simulink model "MagLev_1DOF_Slice_with_noise"  (R2020b)
settings: Solver=ode45  StartTime=0.0  StopTime=15  FixedStep=1e-5  RelTol=1e-3
values from neighbouring files (symbols this model uses):
  c = 0.005    [setup.m]
  caseNumber = 2    [setup.m]
  chi_0 = 0    [setup.m]
  dY_0 = 0.5    [setup.m]
  epsilon = 1e-3    (= 0.001)    [setup.m]
  eth10 = 0.0001    [setup.m]
  g = 9.81    [setup.m]
  gamma_ALCOS = 1000    [setup.m]
  gamma_s = 10    [setup.m]
  gamma_SLICE = 100    [setup.m]
  gamma_y = 10    [setup.m]
  k = 1    [setup.m]
  k0 = kk^3    (= 1000)    [setup.m]
  k1 = 3*kk^2    (= 300)    [setup.m]
  k2 = 3*kk    (= 30)    [setup.m]
  lambda_0 = -0.02    [setup.m]
  m = 0.0844    [setup.m]
  mu = 10    [setup.m]
  nu = 1    [setup.m]
  Omega = [ ... (first row only)    [setup.m]
  R = 2.52    [setup.m]
  s = [1; 2; 10; 20; 5; 7]    [setup.m]
  tt1 = 1    [setup.m]
  tt2 = 3    [setup.m]
  tt3 = 5    [setup.m]
  tt4 = 7    [setup.m]
  Y_0 = -1    [setup.m]
(part 1 of 2)
settings Model: Creator=Alexey  LastModifiedBy=Sviat
settings DataIOCC: ReturnWorkspaceOutputs=off
settings DebuggingCC: ArithmeticOperatorsInVariantConditions=warning
settings SFSimCC: SimUseLocalCustomCode=off  CustomCodeUndefinedFunction=UseInterfaceOnly
settings RTWCC: RTWUseLocalCustomCode=off
settings CodeAppCC: StateflowObjectComments=on

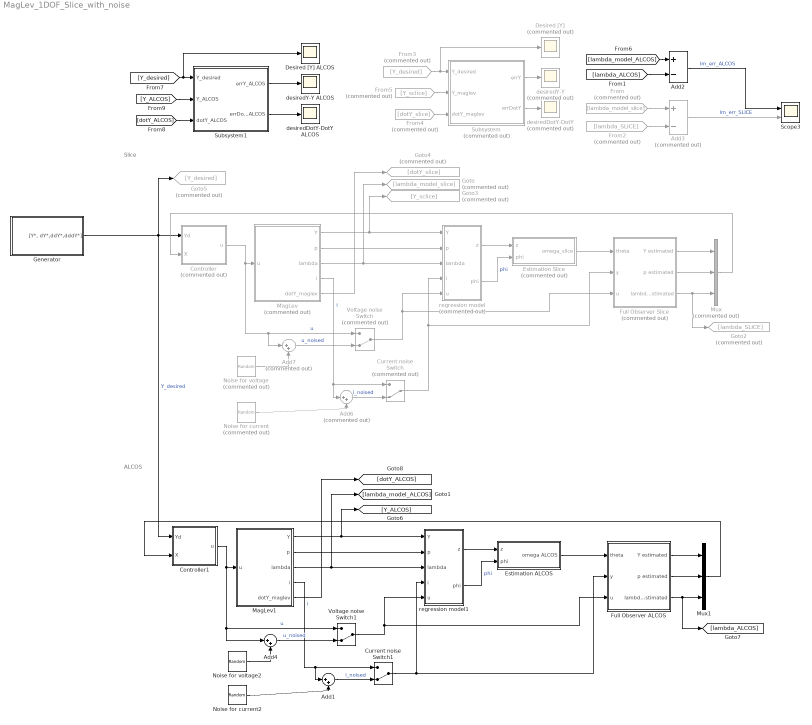
== system MagLev_1DOF_Slice_with_noise ==
  note: Slice
  note: ALCOS
  Add1 : Sum  Inputs=|++
  Add2 : Sum  Inputs=+-
  Add3 : Sum  Commented=on  Inputs=+-
  Add4 : Sum  Inputs=|++
  Add6 : Sum  Commented=on  Inputs=|++
  Add7 : Sum  Commented=on  Inputs=|++
  Controller : MATLAB Function  Commented=on  TreatAsAtomicUnit=on
  Controller1 : MATLAB Function  TreatAsAtomicUnit=on
  Current noise Switch : ManualSwitch  Commented=on  CurrentSetting=0
  Current noise Switch1 : ManualSwitch  CurrentSetting=0
  Desired [Y] : Scope  Commented=on
  Desired [Y] ALCOS : Scope
  Estimation ALCOS : Subsystem
  Estimation Slice : Subsystem  Commented=on
  From : From  Commented=on  GotoTag=lambda_model_slice
  From2 : From  Commented=on  GotoTag=lambda_SLICE
  From3 : From  Commented=on  GotoTag=Y_desired
  From4 : From  Commented=on  GotoTag=dotY_slice
  From5 : From  Commented=on  GotoTag=Y_sclice
  Full Observer ALCOS : Subsystem
  Full Observer Slice : Subsystem  Commented=on
  Generator : Subsystem
  Goto : Goto  Commented=on  GotoTag=lambda_model_slice
  Goto2 : Goto  Commented=on  GotoTag=lambda_SLICE
  Goto3 : Goto  Commented=on  GotoTag=Y_sclice
  Goto4 : Goto  Commented=on  GotoTag=dotY_slice
  Goto5 : Goto  Commented=on  GotoTag=Y_desired
  MagLev : Subsystem  Commented=on
  MagLev1 : Subsystem
  Mux : Mux  Commented=on  Inputs=3
  Mux1 : Mux  Inputs=3
  Noise for current : UniformRandomNumber  Commented=on  Minimum=-0.01  Maximum=0.01  SampleTime=0.0001
  Noise for current2 : UniformRandomNumber  Minimum=-0.01  Maximum=0.01  SampleTime=0.0001
  Noise for voltage : UniformRandomNumber  Commented=on  Minimum=-0.1  Maximum=0.1  SampleTime=0.0001
  Noise for voltage2 : UniformRandomNumber  Minimum=-0.1  Maximum=0.1  SampleTime=0.0001
  Scope3 : Scope  NumInputPorts=2
  Subsystem : Subsystem  Commented=on
  Subsystem1 : Subsystem
  Voltage noise Switch : ManualSwitch  Commented=on  CurrentSetting=0
  Voltage noise Switch1 : ManualSwitch  CurrentSetting=0
  desiredDotY-DotY : Scope  Commented=on
  desiredDotY-DotY ALCOS : Scope
  desiredY-Y : Scope  Commented=on
  desiredY-Y ALCOS : Scope
  regression model : Subsystem  Commented=on
  regression model1 : Subsystem
  wires:
  Controller/1(u) -> MagLev/1(u), Add7/1, Voltage noise Switch/1  "u"
  regression model/2(phi) -> Estimation Slice/2(phi)  "phi"
  regression model/1(z) -> Estimation Slice/1(z)
  MagLev/4(i) -> Add6/1, Current noise Switch/1  "i"
  Estimation Slice/1(omega_slice) -> Full Observer Slice/1(theta)
  From/1 -> Add3/1
  [lambda_ALCOS] -> Add2/2
  From2/1 -> Add3/2
  Add3/1 -> Scope3/2  "lm_err_SLICE"
  Current noise Switch/1 -> Full Observer Slice/2(y), regression model/4(i)
  Noise for voltage/1 -> Add7/2
  Noise for current/1 -> Add6/2
  Add6/1 -> Current noise Switch/2  "i_noised"
  Add7/1 -> Voltage noise Switch/2  "u_noised"
  Voltage noise Switch/1 -> Full Observer Slice/3(u), regression model/5(u)
  Subsystem/1(errY) -> desiredY-Y/1
  Subsystem/2(errDotY) -> desiredDotY-DotY/1
  From3/1 -> Desired [Y]/1, Subsystem/1(Y_desired)
  MagLev/1(Y) -> Goto3/1, regression model/1(Y)
  MagLev/2(p) -> regression model/2(p)
  MagLev/3(lambda) -> regression model/3(lambda), Goto/1
  MagLev/5(dotY_maglev) -> Goto4/1
  MagLev1/2(p) -> regression model1/2(p)
  MagLev1/1(Y) -> [Y_ALCOS], regression model1/1(Y)
  Voltage noise Switch1/1 -> Full Observer ALCOS/3(u), regression model1/5(u)
  Add1/1 -> Current noise Switch1/2  "i_noised"
  Noise for voltage2/1 -> Add4/2
  Controller1/1(u) -> MagLev1/1(u), Voltage noise Switch1/1, Add4/1  "u"
  Generator/1("[Y*, dY*,ddY*,dddY*]") -> Goto5/1, Controller/1(Yd), Controller1/1(Yd)  "Y_desired"
  MagLev1/4(i) -> Add1/1, Current noise Switch1/1  "i"
  Current noise Switch1/1 -> Full Observer ALCOS/2(y), regression model1/4(i)
  regression model1/2(phi) -> Estimation ALCOS/2(phi)  "phi"
  regression model1/1(z) -> Estimation ALCOS/1(z)
  Estimation ALCOS/1(omega ALCOS) -> Full Observer ALCOS/1(theta)
  Add4/1 -> Voltage noise Switch1/2  "u_noised"
  MagLev1/3(lambda) -> [lambda_model_ALCOS], regression model1/3(lambda)
  Full Observer Slice/1(Y estimated) -> Mux/1
  Full Observer Slice/2(p estimated) -> Mux/2
  Full Observer Slice/3(lambda estimated) -> Goto2/1, Mux/3
  Full Observer ALCOS/1(Y estimated) -> Mux1/1
  Full Observer ALCOS/2(p estimated) -> Mux1/2
  From5/1 -> Subsystem/2(Y_maglev)
  From4/1 -> Subsystem/3(dotY_maglev)
  Add2/1 -> Scope3/1  "lm_err_ALCOS"
  Noise for current2/1 -> Add1/2
  Mux/1 -> Controller/2(X)
  Full Observer ALCOS/3(lambda estimated) -> [lambda_ALCOS], Mux1/3
  Mux1/1 -> Controller1/2(X)
  [lambda_model_ALCOS] -> Add2/1
  MagLev1/5(dotY_maglev) -> [dotY_ALCOS]
  [dotY_ALCOS] -> Subsystem1/3(dotY_ALCOS)
  [Y_ALCOS] -> Subsystem1/2(Y_ALCOS)
  [Y_desired] -> Desired [Y] ALCOS/1, Subsystem1/1(Y_desired)
  Subsystem1/2(errDotY_ALCOS) -> desiredDotY-DotY ALCOS/1
  Subsystem1/1(errY_ALCOS) -> desiredY-Y ALCOS/1

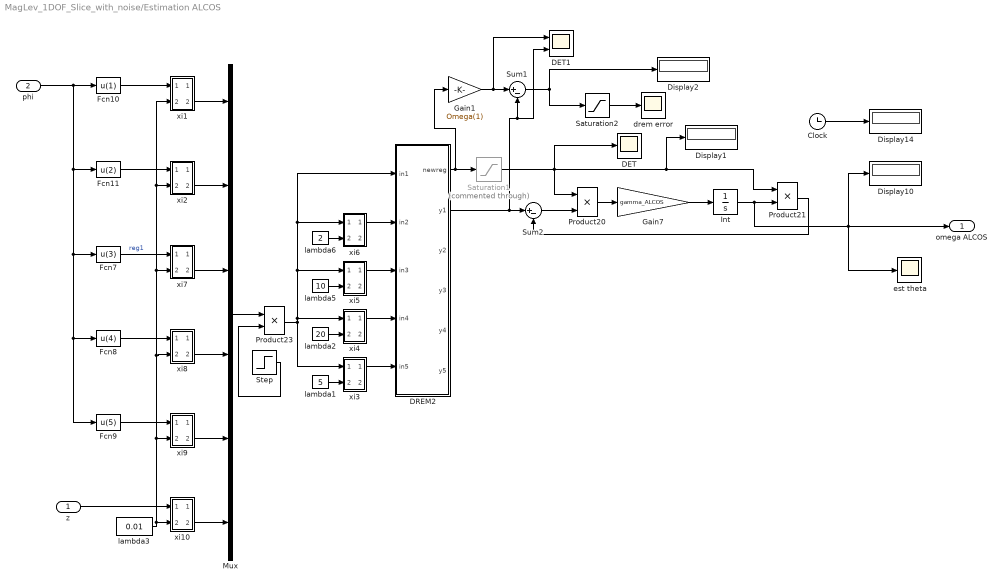
== system MagLev_1DOF_Slice_with_noise/Estimation ALCOS ==
  z : Inport
  phi : Inport  Port=2
  Clock : Clock
  DET : Scope
  DET1 : Scope  NumInputPorts=2
  DREM2 : MATLAB Function  TreatAsAtomicUnit=on
  Display{1..2,10,14} (4 alike) : Display
  Fcn10 : Fcn  Expr=u(1)
  Fcn11 : Fcn  Expr=u(2)
  Fcn7 : Fcn  Expr=u(3)
  Fcn8 : Fcn  Expr=u(4)
  Fcn9 : Fcn  Expr=u(5)
  Gain1 : Gain  Gain=Omega(1)
  Gain7 : Gain  Gain=gamma_ALCOS
  Int : Integrator  InitialCondition=eth10
  Mux : Mux  Inputs=6
  Product20 : Product  RndMeth=Zero
  Product21 : Product  RndMeth=Zero
  Product23 : Product  RndMeth=Zero
  Saturation1 : Saturate  Commented=through  UpperLimit=1000  LowerLimit=-1000
  Saturation2 : Saturate  UpperLimit=1000  LowerLimit=-1000
  Step : Step  Time=0  After=100  SampleTime=0
  Sum1 : Sum  Inputs=|+-
  Sum2 : Sum  Inputs=|+-
  drem error : Scope
  est theta : Scope
  lambda1 : Constant  Value=5
  lambda2 : Constant  Value=20
  lambda3 : Constant  Value=0.01
  lambda5 : Constant  Value=10
  lambda6 : Constant  Value=2
  xi1 : Subsystem
  xi10 : Subsystem
  xi2 : Subsystem
  xi3 : Subsystem
  xi4 : Subsystem
  xi5 : Subsystem
  xi6 : Subsystem
  xi7 : Subsystem
  xi8 : Subsystem
  xi9 : Subsystem
  omega ALCOS : Outport  VectorParamsAs1DForOutWhenUnconnected=off
  wires:
  Mux/1 -> Product23/1
  Product20/1 -> Gain7/1
  Gain7/1 -> Int/1
  Int/1 -> omega ALCOS/1, est theta/1, Display10/1, Product21/2
  Product21/1 -> Sum2/2
  Sum2/1 -> Product20/2
  DREM2/2(y1) -> Sum2/1, DET1/2, Sum1/2
  Clock/1 -> Display14/1
  DREM2/1(newreg) -> Saturation1/1, Gain1/1
  Product23/1 -> DREM2/1(in1), xi6/1(Input), xi5/1(Input), xi4/1(Input), xi3/1(Input)
  lambda1/1 -> xi3/2(lambda)
  xi3/1(Output) -> DREM2/5(in5)
  lambda2/1 -> xi4/2(lambda)
  lambda5/1 -> xi5/2(lambda)
  lambda6/1 -> xi6/2(lambda)
  xi6/1(Output) -> DREM2/2(in2)
  xi5/1(Output) -> DREM2/3(in3)
  xi4/1(Output) -> DREM2/4(in4)
  Fcn9/1 -> xi9/1(Input)
  Fcn8/1 -> xi8/1(Input)
  Fcn7/1 -> xi7/1(Input)  "reg1"
  Fcn11/1 -> xi2/1(Input)
  Fcn10/1 -> xi1/1(Input)
  xi1/2(Output1) -> Mux/1
  xi2/2(Output1) -> Mux/2
  xi7/2(Output1) -> Mux/3
  xi8/2(Output1) -> Mux/4
  xi9/2(Output1) -> Mux/5
  xi10/2(Output1) -> Mux/6
  lambda3/1 -> xi8/2(lambda), xi7/2(lambda), xi1/2(lambda), xi2/2(lambda), xi9/2(lambda), xi10/2(lambda)
  Step/1 -> Product23/2
  Saturation1/1 -> DET/1, Product20/1, Display1/1, Product21/1
  z/1 -> xi10/1(Input)
  phi/1 -> Fcn9/1, Fcn8/1, Fcn7/1, Fcn11/1, Fcn10/1
  Gain1/1 -> DET1/1, Sum1/1
  Sum1/1 -> Display2/1, Saturation2/1
  Saturation2/1 -> drem error/1

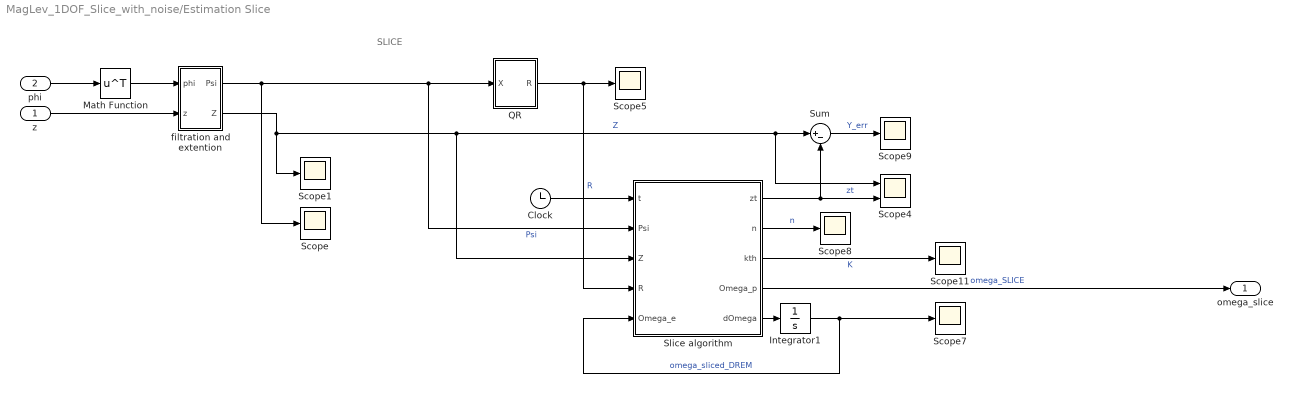
== system MagLev_1DOF_Slice_with_noise/Estimation Slice ==
  note: SLICE
  z : Inport
  phi : Inport  Port=2
  Clock : Clock
  Integrator1 : Integrator  InitialCondition=eth10
  Math Function : Math  Operator=transpose  SignedPower=on  SaturateOnIntegerOverflow=on
  QR : MATLAB Function  TreatAsAtomicUnit=on
  Scope{,1,5,7..9,11} (7 alike) : Scope
  Scope4 : Scope  NumInputPorts=2
  Slice algorithm : MATLAB Function  TreatAsAtomicUnit=on
  Sum : Sum  Inputs=|+-
  filtration and extention : Subsystem
  omega_slice : Outport  VectorParamsAs1DForOutWhenUnconnected=off
  wires:
  z/1 -> filtration and extention/2(z)
  phi/1 -> Math Function/1
  filtration and extention/1(Psi) -> Slice algorithm/2(Psi), QR/1(X), Scope/1  "Psi"
  filtration and extention/2(Z) -> Sum/1, Scope4/1, Slice algorithm/3(Z), Scope1/1  "Z"
  Math Function/1 -> filtration and extention/1(phi)
  Slice algorithm/5(dOmega) -> Integrator1/1
  QR/1(R) -> Scope5/1, Slice algorithm/4(R)  "R"
  Integrator1/1 -> Scope7/1, Slice algorithm/5(Omega_e)  "omega_sliced_DREM"
  Slice algorithm/4(Omega_p) -> omega_slice/1  "omega_SLICE"
  Slice algorithm/1(zt) -> Scope4/2, Sum/2  "zt"
  Slice algorithm/2(n) -> Scope8/1  "n"
  Sum/1 -> Scope9/1  "Y_err"
  Slice algorithm/3(kth) -> Scope11/1  "K"
  Clock/1 -> Slice algorithm/1(t)

== system MagLev_1DOF_Slice_with_noise/Full Observer ALCOS ==
  theta : Inport
  y : Inport  Port=2
  u : Inport  Port=3
  Flux Observer : Subsystem
  Gain1 : Gain  Gain=m
  Position Observer : Subsystem
  Speed Observer : Subsystem
  est Y : Scope
  est dY : Scope
  est lambda : Scope
  Y estimated : Outport  VectorParamsAs1DForOutWhenUnconnected=off
  p estimated : Outport  Port=2  VectorParamsAs1DForOutWhenUnconnected=off
  lambda estimated : Outport  Port=3  VectorParamsAs1DForOutWhenUnconnected=off
  wires:
  Flux Observer/1("lambda ") -> est lambda/1, Position Observer/1(lambda), lambda estimated/1, Speed Observer/1(lambda)
  Speed Observer/1(dY) -> est dY/1, Position Observer/3(v), Gain1/1
  theta/1 -> Flux Observer/1(theta)
  y/1 -> Position Observer/2(I), Speed Observer/2(I), Flux Observer/2(I)
  u/1 -> Speed Observer/3(u), Flux Observer/3(u)
  Position Observer/1(Y) -> est Y/1, Y estimated/1
  Gain1/1 -> p estimated/1

== system MagLev_1DOF_Slice_with_noise/Full Observer Slice ==
  theta : Inport
  y : Inport  Port=2
  u : Inport  Port=3
  Flux Observer : Subsystem
  Gain1 : Gain  Gain=m
  Position Observer : Subsystem
  Speed Observer : Subsystem
  Y estimated : Outport  VectorParamsAs1DForOutWhenUnconnected=off
  p estimated : Outport  Port=2  VectorParamsAs1DForOutWhenUnconnected=off
  lambda estimated : Outport  Port=3  VectorParamsAs1DForOutWhenUnconnected=off
  wires:
  Speed Observer/1(dY) -> Position Observer/3(v), Gain1/1
  theta/1 -> Flux Observer/1(theta)
  y/1 -> Position Observer/2(I), Speed Observer/2(I), Flux Observer/2(I)
  u/1 -> Speed Observer/3(u), Flux Observer/3(u)
  Position Observer/1(Y) -> Y estimated/1
  Gain1/1 -> p estimated/1
  Flux Observer/1("lambda ") -> Position Observer/1(lambda), lambda estimated/1, Speed Observer/1(lambda)

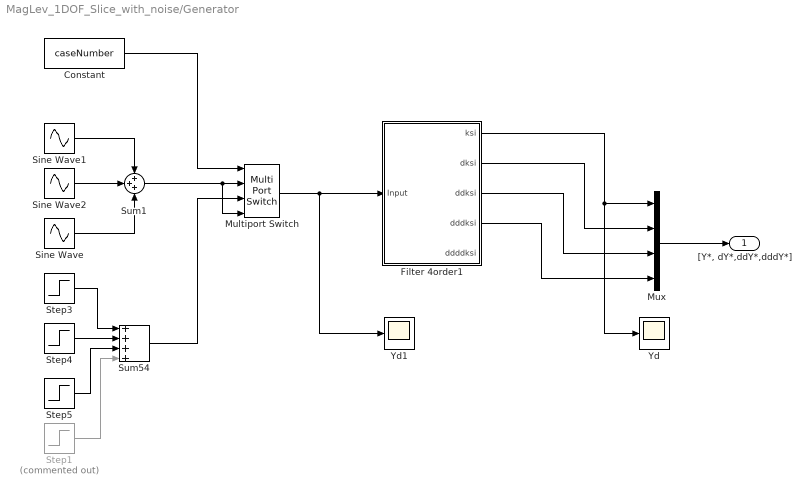
== system MagLev_1DOF_Slice_with_noise/Generator ==
  Constant : Constant  Value=caseNumber
  Filter 4order1 : Subsystem
  Multiport Switch : MultiPortSwitch
  Mux : Mux
  Sine Wave : Sin  SampleTime=0
  Sine Wave1 : Sin  Amplitude=0.5  Frequency=3.7  Phase=pi/3  SampleTime=0
  Sine Wave2 : Sin  Frequency=2  SampleTime=0
  Step1 : Step  Commented=on  Time=tt4  After=-1  SampleTime=0
  Step3 : Step  Time=tt1  After=2  SampleTime=0
  Step4 : Step  Time=tt2  After=-2  SampleTime=0
  Step5 : Step  Time=tt3  After=3  SampleTime=0
  Sum1 : Sum  Inputs=+++
  Sum54 : Sum  Inputs=++++
  Yd : Scope
  Yd1 : Scope
  "[Y*, dY*,ddY*,dddY*]" : Outport  VectorParamsAs1DForOutWhenUnconnected=off
  wires:
  Mux/1 -> "[Y*, dY*,ddY*,dddY*]"/1
  Filter 4order1/1(ksi) -> Yd/1, Mux/1
  Filter 4order1/2(dksi) -> Mux/2
  Filter 4order1/3(ddksi) -> Mux/3
  Filter 4order1/4(dddksi) -> Mux/4
  Step3/1 -> Sum54/1
  Step4/1 -> Sum54/2
  Step5/1 -> Sum54/3
  Step1/1 -> Sum54/4
  Constant/1 -> Multiport Switch/1
  Sum1/1 -> Multiport Switch/4, Multiport Switch/2
  Sum54/1 -> Multiport Switch/3
  Sine Wave/1 -> Sum1/3
  Sine Wave2/1 -> Sum1/2
  Sine Wave1/1 -> Sum1/1
  Multiport Switch/1 -> Yd1/1, Filter 4order1/1(Input)

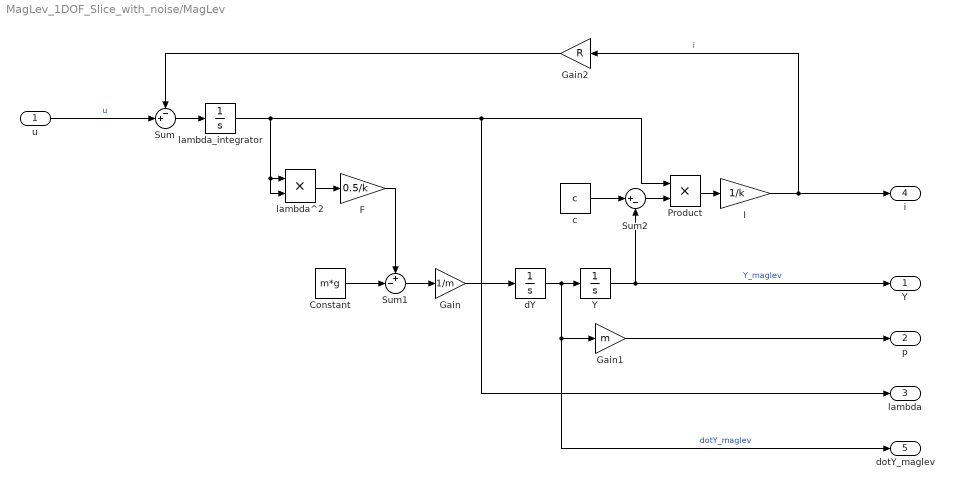
== system MagLev_1DOF_Slice_with_noise/MagLev ==
  u : Inport
  " I " : Gain  Gain=1/k
  Constant : Constant  Value=m*g
  "F " : Gain  Gain=0.5/k
  Gain : Gain  Gain=1/m
  Gain1 : Gain  Gain=m
  Gain2 : Gain  Gain=R
  Product : Product
  Sum : Sum  Inputs=-+|
  Sum1 : Sum  Inputs=+-|
  Sum2 : Sum  Inputs=|+-
  "Y " : Integrator  InitialCondition=Y_0
  c : Constant  Value=c
  dY : Integrator  InitialCondition=dY_0
  lambda^2 : Product
  lambda_integrator : Integrator  InitialCondition=lambda_0
  Y : Outport  PortDimensions=1  VectorParamsAs1DForOutWhenUnconnected=off
  p : Outport  Port=2  PortDimensions=1  VectorParamsAs1DForOutWhenUnconnected=off
  lambda : Outport  Port=3  PortDimensions=1  VectorParamsAs1DForOutWhenUnconnected=off
  i : Outport  Port=4  PortDimensions=1  VectorParamsAs1DForOutWhenUnconnected=off
  dotY_maglev : Outport  Port=5  PortDimensions=1  VectorParamsAs1DForOutWhenUnconnected=off
  wires:
  Sum/1 -> lambda_integrator/1
  dY/1 -> dotY_maglev/1, Gain1/1, "Y "/1  "dotY_maglev"
  Gain/1 -> dY/1
  Sum1/1 -> Gain/1
  Constant/1 -> Sum1/2
  c/1 -> Sum2/1
  Sum2/1 -> Product/2
  lambda_integrator/1 -> lambda/1, Product/1, lambda^2/2, lambda^2/1
  Product/1 -> " I "/1
  lambda^2/1 -> "F "/1
  "F "/1 -> Sum1/1
  Gain2/1 -> Sum/1
  "Y "/1 -> Y/1, Sum2/2  "Y_maglev"
  Gain1/1 -> p/1
  u/1 -> Sum/2  "u"
  " I "/1 -> i/1, Gain2/1  "i"

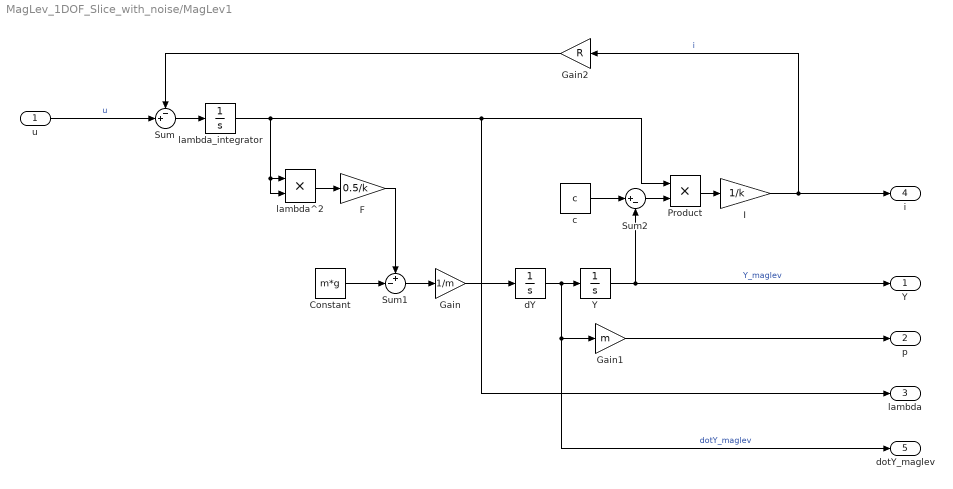
== system MagLev_1DOF_Slice_with_noise/MagLev1 ==
  u : Inport
  " I " : Gain  Gain=1/k
  Constant : Constant  Value=m*g
  "F " : Gain  Gain=0.5/k
  Gain : Gain  Gain=1/m
  Gain1 : Gain  Gain=m
  Gain2 : Gain  Gain=R
  Product : Product
  Sum : Sum  Inputs=-+|
  Sum1 : Sum  Inputs=+-|
  Sum2 : Sum  Inputs=|+-
  "Y " : Integrator  InitialCondition=Y_0
  c : Constant  Value=c
  dY : Integrator  InitialCondition=dY_0
  lambda^2 : Product
  lambda_integrator : Integrator  InitialCondition=lambda_0
  Y : Outport  PortDimensions=1  VectorParamsAs1DForOutWhenUnconnected=off
  p : Outport  Port=2  PortDimensions=1  VectorParamsAs1DForOutWhenUnconnected=off
  lambda : Outport  Port=3  PortDimensions=1  VectorParamsAs1DForOutWhenUnconnected=off
  i : Outport  Port=4  PortDimensions=1  VectorParamsAs1DForOutWhenUnconnected=off
  dotY_maglev : Outport  Port=5  PortDimensions=1  VectorParamsAs1DForOutWhenUnconnected=off
  wires:
  Sum/1 -> lambda_integrator/1
  Gain/1 -> dY/1
  Sum1/1 -> Gain/1
  Constant/1 -> Sum1/2
  c/1 -> Sum2/1
  Sum2/1 -> Product/2
  lambda_integrator/1 -> lambda/1, Product/1, lambda^2/2, lambda^2/1
  Product/1 -> " I "/1
  lambda^2/1 -> "F "/1
  "F "/1 -> Sum1/1
  Gain2/1 -> Sum/1
  "Y "/1 -> Y/1, Sum2/2  "Y_maglev"
  Gain1/1 -> p/1
  u/1 -> Sum/2  "u"
  " I "/1 -> i/1, Gain2/1  "i"
  dY/1 -> dotY_maglev/1, Gain1/1, "Y "/1  "dotY_maglev"

== system MagLev_1DOF_Slice_with_noise/Subsystem ==
  Y_desired : Inport
  Y_maglev : Inport  Port=2  PortDimensions=1
  dotY_maglev : Inport  Port=3  PortDimensions=1
  Add4 : Sum  Inputs=+-
  Add5 : Sum  Inputs=+-
  Demux1 : Demux
  Y_diff : Scope  NumInputPorts=3
  desiredY-Y : Scope  NumInputPorts=2
  errY : Outport
  errDotY : Outport  Port=2
  wires:
  Y_maglev/1 -> Y_diff/1, desiredY-Y/2, Add4/2
  dotY_maglev/1 -> Add5/2, Y_diff/2
  Y_desired/1 -> Demux1/1, Y_diff/3
  Add4/1 -> errY/1  "errY"
  Demux1/2 -> Add5/1
  Demux1/1 -> desiredY-Y/1, Add4/1  "Y"
  Add5/1 -> errDotY/1  "errDotY"

== system MagLev_1DOF_Slice_with_noise/Subsystem1 ==
  Y_desired : Inport
  Y_ALCOS : Inport  Port=2  PortDimensions=1
  dotY_ALCOS : Inport  Port=3  PortDimensions=1
  Add4 : Sum  Inputs=+-
  Add5 : Sum  Inputs=+-
  Demux1 : Demux
  errY_ALCOS : Outport
  errDotY_ALCOS : Outport  Port=2
  wires:
  Y_ALCOS/1 -> Add4/2
  dotY_ALCOS/1 -> Add5/2
  Y_desired/1 -> Demux1/1
  Add4/1 -> errY_ALCOS/1  "errY_ALCOS"
  Demux1/2 -> Add5/1
  Demux1/1 -> Add4/1  "Y"
  Add5/1 -> errDotY_ALCOS/1  "errDotY_ALCOS"

== system MagLev_1DOF_Slice_with_noise/regression model ==
  Y : Inport
  p : Inport  Port=2
  lambda : Inport  Port=3
  i : Inport  Port=4
  u : Inport  Port=5
  "  regression model" : Subsystem
  Vectorize : Subsystem
  z : Outport  VectorParamsAs1DForOutWhenUnconnected=off
  phi : Outport  Port=2  VectorParamsAs1DForOutWhenUnconnected=off
  wires:
  u/1 -> Vectorize/5(u)  "u"
  Vectorize/1(v) -> "  regression model"/1(v)
  "  regression model"/1(z) -> z/1
  "  regression model"/2(phi) -> phi/1
  p/1 -> Vectorize/2(x2)  "p"
  lambda/1 -> Vectorize/3(x3)  "lambda"
  i/1 -> Vectorize/4(y)  "i"
  Y/1 -> Vectorize/1(x1)  "Y"

== system MagLev_1DOF_Slice_with_noise/regression model1 ==
  Y : Inport
  p : Inport  Port=2
  lambda : Inport  Port=3
  i : Inport  Port=4
  u : Inport  Port=5
  "  regression model" : Subsystem
  Vectorize : Subsystem
  z : Outport  VectorParamsAs1DForOutWhenUnconnected=off
  phi : Outport  Port=2  VectorParamsAs1DForOutWhenUnconnected=off
  wires:
  u/1 -> Vectorize/5(u)  "u"
  Vectorize/1(v) -> "  regression model"/1(v)
  "  regression model"/1(z) -> z/1
  "  regression model"/2(phi) -> phi/1
  p/1 -> Vectorize/2(x2)  "p"
  lambda/1 -> Vectorize/3(x3)  "lambda"
  i/1 -> Vectorize/4(y)  "i"
  Y/1 -> Vectorize/1(x1)  "Y"

== system MagLev_1DOF_Slice_with_noise/Estimation ALCOS/xi1 ==
  Input : Inport
  lambda : Inport  Port=2
  Int : Integrator
  Product : Product  RndMeth=Zero
  Sum1 : Sum  Inputs=|+-
  Output : Outport  VectorParamsAs1DForOutWhenUnconnected=off
  Output1 : Outport  Port=2  VectorParamsAs1DForOutWhenUnconnected=off
  wires:
  Input/1 -> Sum1/1
  lambda/1 -> Product/2
  Int/1 -> Sum1/2, Output/1
  Product/1 -> Output1/1, Int/1
  Sum1/1 -> Product/1

== system MagLev_1DOF_Slice_with_noise/Estimation ALCOS/xi10 ==
  Input : Inport
  lambda : Inport  Port=2
  Int : Integrator
  Product : Product  RndMeth=Zero
  Sum1 : Sum  Inputs=|+-
  Output : Outport  VectorParamsAs1DForOutWhenUnconnected=off
  Output1 : Outport  Port=2  VectorParamsAs1DForOutWhenUnconnected=off
  wires:
  Input/1 -> Sum1/1
  lambda/1 -> Product/2
  Int/1 -> Sum1/2, Output/1
  Product/1 -> Output1/1, Int/1
  Sum1/1 -> Product/1

== system MagLev_1DOF_Slice_with_noise/Estimation ALCOS/xi2 ==
  Input : Inport
  lambda : Inport  Port=2
  Int : Integrator
  Product : Product  RndMeth=Zero
  Sum1 : Sum  Inputs=|+-
  Output : Outport  VectorParamsAs1DForOutWhenUnconnected=off
  Output1 : Outport  Port=2  VectorParamsAs1DForOutWhenUnconnected=off
  wires:
  Sum1/1 -> Product/1
  Product/1 -> Int/1, Output1/1
  Int/1 -> Output/1, Sum1/2
  lambda/1 -> Product/2
  Input/1 -> Sum1/1

== system MagLev_1DOF_Slice_with_noise/Estimation ALCOS/xi3 ==
  Input : Inport
  lambda : Inport  Port=2
  Int : Integrator
  Product : Product  RndMeth=Zero
  Sum1 : Sum  Inputs=|+-
  Output : Outport  VectorParamsAs1DForOutWhenUnconnected=off
  Output1 : Outport  Port=2  VectorParamsAs1DForOutWhenUnconnected=off
  wires:
  Input/1 -> Sum1/1
  lambda/1 -> Product/2
  Int/1 -> Sum1/2, Output/1
  Product/1 -> Output1/1, Int/1
  Sum1/1 -> Product/1

== system MagLev_1DOF_Slice_with_noise/Estimation ALCOS/xi4 ==
  Input : Inport
  lambda : Inport  Port=2
  Int : Integrator
  Product : Product  RndMeth=Zero
  Sum1 : Sum  Inputs=|+-
  Output : Outport  VectorParamsAs1DForOutWhenUnconnected=off
  Output1 : Outport  Port=2  VectorParamsAs1DForOutWhenUnconnected=off
  wires:
  Sum1/1 -> Product/1
  Product/1 -> Int/1, Output1/1
  Int/1 -> Output/1, Sum1/2
  lambda/1 -> Product/2
  Input/1 -> Sum1/1

== system MagLev_1DOF_Slice_with_noise/Estimation ALCOS/xi5 ==
  Input : Inport
  lambda : Inport  Port=2
  Int : Integrator
  Product : Product  RndMeth=Zero
  Sum1 : Sum  Inputs=|+-
  Output : Outport  VectorParamsAs1DForOutWhenUnconnected=off
  Output1 : Outport  Port=2  VectorParamsAs1DForOutWhenUnconnected=off
  wires:
  Input/1 -> Sum1/1
  lambda/1 -> Product/2
  Int/1 -> Sum1/2, Output/1
  Product/1 -> Output1/1, Int/1
  Sum1/1 -> Product/1

== system MagLev_1DOF_Slice_with_noise/Estimation ALCOS/xi6 ==
  Input : Inport
  lambda : Inport  Port=2
  Int : Integrator
  Product : Product  RndMeth=Zero
  Sum1 : Sum  Inputs=|+-
  Output : Outport  VectorParamsAs1DForOutWhenUnconnected=off
  Output1 : Outport  Port=2  VectorParamsAs1DForOutWhenUnconnected=off
  wires:
  Sum1/1 -> Product/1
  Product/1 -> Int/1, Output1/1
  Int/1 -> Output/1, Sum1/2
  lambda/1 -> Product/2
  Input/1 -> Sum1/1

== system MagLev_1DOF_Slice_with_noise/Estimation ALCOS/xi7 ==
  Input : Inport
  lambda : Inport  Port=2
  Int : Integrator
  Product : Product  RndMeth=Zero
  Sum1 : Sum  Inputs=|+-
  Output : Outport  VectorParamsAs1DForOutWhenUnconnected=off
  Output1 : Outport  Port=2  VectorParamsAs1DForOutWhenUnconnected=off
  wires:
  Sum1/1 -> Product/1
  Product/1 -> Int/1, Output1/1
  Int/1 -> Output/1, Sum1/2
  lambda/1 -> Product/2
  Input/1 -> Sum1/1

== system MagLev_1DOF_Slice_with_noise/Estimation ALCOS/xi8 ==
  Input : Inport
  lambda : Inport  Port=2
  Int : Integrator
  Product : Product  RndMeth=Zero
  Sum1 : Sum  Inputs=|+-
  Output : Outport  VectorParamsAs1DForOutWhenUnconnected=off
  Output1 : Outport  Port=2  VectorParamsAs1DForOutWhenUnconnected=off
  wires:
  Input/1 -> Sum1/1
  lambda/1 -> Product/2
  Int/1 -> Sum1/2, Output/1
  Product/1 -> Output1/1, Int/1
  Sum1/1 -> Product/1

== system MagLev_1DOF_Slice_with_noise/Estimation ALCOS/xi9 ==
  Input : Inport
  lambda : Inport  Port=2
  Int : Integrator
  Product : Product  RndMeth=Zero
  Sum1 : Sum  Inputs=|+-
  Output : Outport  VectorParamsAs1DForOutWhenUnconnected=off
  Output1 : Outport  Port=2  VectorParamsAs1DForOutWhenUnconnected=off
  wires:
  Sum1/1 -> Product/1
  Product/1 -> Int/1, Output1/1
  Int/1 -> Output/1, Sum1/2
  lambda/1 -> Product/2
  Input/1 -> Sum1/1

== system MagLev_1DOF_Slice_with_noise/Estimation Slice/filtration and extention ==
  note: Regressor filtration
  note: Output filtration
  phi : Inport
  z : Inport  Port=2
  Gain : Gain  Gain=diag(s)  Multiplication=Matrix(K*u)
  Gain1 : Gain  Gain=s  Multiplication=Matrix(K*u)
  Gain2 : Gain  Gain=s  Multiplication=Matrix(K*u)
  Gain3 : Gain  Gain=diag(s)  Multiplication=Matrix(K*u)
  Integrator : Integrator
  Integrator1 : Integrator
  Sum : Sum  Inputs=|+-
  Sum1 : Sum  Inputs=|+-
  Psi : Outport  VectorParamsAs1DForOutWhenUnconnected=off
  Z : Outport  Port=2  VectorParamsAs1DForOutWhenUnconnected=off
  wires:
  Gain/1 -> Sum/2
  phi/1 -> Gain1/1  "phi"
  Integrator/1 -> Psi/1, Gain/1  "Psi"
  Gain3/1 -> Sum1/2
  Gain1/1 -> Sum/1
  Sum1/1 -> Integrator1/1
  Integrator1/1 -> Z/1, Gain3/1  "Z"
  Sum/1 -> Integrator/1
  z/1 -> Gain2/1  "z"
  Gain2/1 -> Sum1/1

== system MagLev_1DOF_Slice_with_noise/Full Observer ALCOS/Flux Observer ==
  theta : Inport
  I : Inport  Port=2
  u : Inport  Port=3
  Gain1 : Gain  Gain=R
  Sum1 : Sum  Inputs=|-+
  Sum5 : Sum  Inputs=++|
  psi : Integrator
  "lambda " : Outport  VectorParamsAs1DForOutWhenUnconnected=off
  wires:
  Sum1/1 -> psi/1
  I/1 -> Gain1/1
  Gain1/1 -> Sum1/1
  u/1 -> Sum1/2
  psi/1 -> Sum5/2
  Sum5/1 -> "lambda "/1
  theta/1 -> Sum5/1

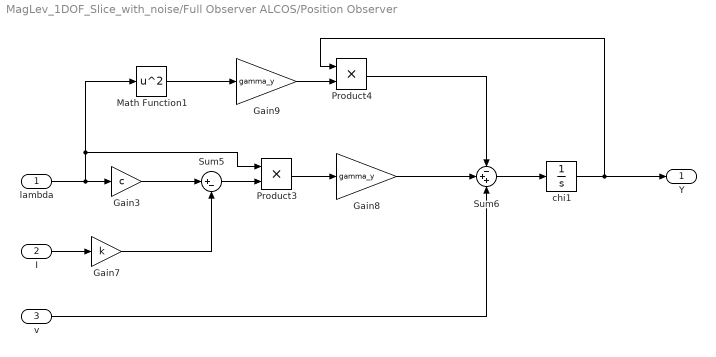
== system MagLev_1DOF_Slice_with_noise/Full Observer ALCOS/Position Observer ==
  lambda : Inport
  I : Inport  Port=2
  v : Inport  Port=3
  Gain3 : Gain  Gain=c
  Gain7 : Gain  Gain=k
  Gain8 : Gain  Gain=gamma_y
  Gain9 : Gain  Gain=gamma_y
  Math Function1 : Math  Operator=square  SignedPower=on  SaturateOnIntegerOverflow=on
  Product3 : Product
  Product4 : Product
  Sum5 : Sum  Inputs=|+-
  Sum6 : Sum  Inputs=-++
  chi1 : Integrator  InitialCondition=chi_0
  Y : Outport  VectorParamsAs1DForOutWhenUnconnected=off
  wires:
  lambda/1 -> Math Function1/1, Product3/1, Gain3/1
  Gain3/1 -> Sum5/1
  I/1 -> Gain7/1
  Gain7/1 -> Sum5/2
  Sum5/1 -> Product3/2
  Product3/1 -> Gain8/1
  Math Function1/1 -> Gain9/1
  Gain9/1 -> Product4/2
  chi1/1 -> Y/1, Product4/1
  Product4/1 -> Sum6/1
  v/1 -> Sum6/3
  Gain8/1 -> Sum6/2
  Sum6/1 -> chi1/1

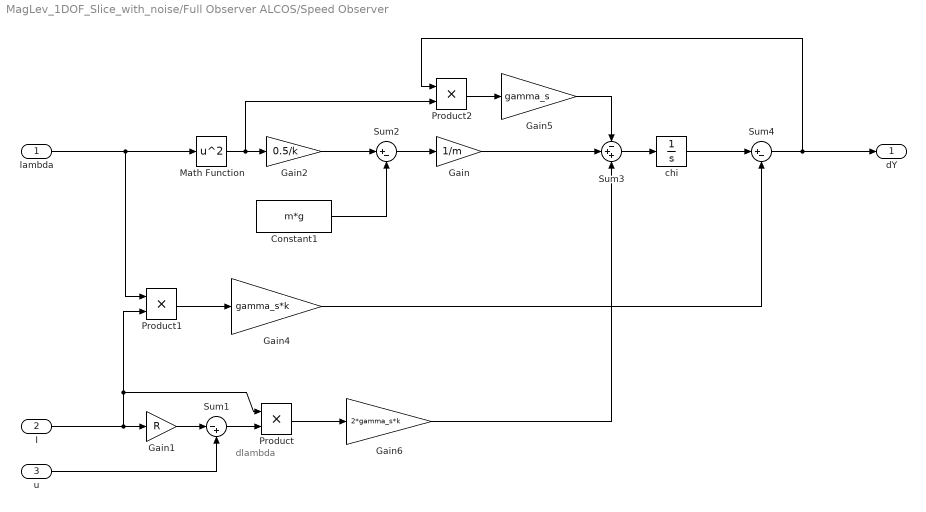
== system MagLev_1DOF_Slice_with_noise/Full Observer ALCOS/Speed Observer ==
  note: dlambda
  lambda : Inport
  I : Inport  Port=2
  u : Inport  Port=3
  Constant1 : Constant  Value=m*g
  Gain : Gain  Gain=1/m
  Gain1 : Gain  Gain=R
  Gain2 : Gain  Gain=0.5/k
  Gain4 : Gain  Gain=gamma_s*k
  Gain5 : Gain  Gain=gamma_s
  Gain6 : Gain  Gain=2*gamma_s*k
  Math Function : Math  Operator=square  SignedPower=on  SaturateOnIntegerOverflow=on
  Product : Product
  Product1 : Product
  Product2 : Product
  Sum1 : Sum  Inputs=|-+
  Sum2 : Sum  Inputs=|+-
  Sum3 : Sum  Inputs=-++
  Sum4 : Sum  Inputs=|+-
  chi : Integrator
  dY : Outport  VectorParamsAs1DForOutWhenUnconnected=off
  wires:
  u/1 -> Sum1/2
  Gain1/1 -> Sum1/1
  I/1 -> Product1/2, Product/1, Gain1/1
  lambda/1 -> Math Function/1, Product1/1
  Math Function/1 -> Product2/2, Gain2/1
  Sum2/1 -> Gain/1
  Sum1/1 -> Product/2
  Product/1 -> Gain6/1
  Sum3/1 -> chi/1
  chi/1 -> Sum4/1
  Product1/1 -> Gain4/1
  Gain4/1 -> Sum4/2
  Sum4/1 -> Product2/1, dY/1
  Gain/1 -> Sum3/2
  Constant1/1 -> Sum2/2
  Gain2/1 -> Sum2/1
  Product2/1 -> Gain5/1
  Gain5/1 -> Sum3/1
  Gain6/1 -> Sum3/3

== system MagLev_1DOF_Slice_with_noise/Full Observer Slice/Flux Observer ==
  theta : Inport
  I : Inport  Port=2
  u : Inport  Port=3
  Gain1 : Gain  Gain=R
  Sum1 : Sum  Inputs=|-+
  Sum5 : Sum  Inputs=++|
  psi : Integrator
  "lambda " : Outport  VectorParamsAs1DForOutWhenUnconnected=off
  wires:
  Sum1/1 -> psi/1
  I/1 -> Gain1/1
  Gain1/1 -> Sum1/1
  u/1 -> Sum1/2
  psi/1 -> Sum5/2
  Sum5/1 -> "lambda "/1
  theta/1 -> Sum5/1

== system MagLev_1DOF_Slice_with_noise/Full Observer Slice/Position Observer ==
  lambda : Inport
  I : Inport  Port=2
  v : Inport  Port=3
  Gain3 : Gain  Gain=c
  Gain7 : Gain  Gain=k
  Gain8 : Gain  Gain=gamma_y
  Gain9 : Gain  Gain=gamma_y
  Math Function1 : Math  Operator=square  SignedPower=on  SaturateOnIntegerOverflow=on
  Product3 : Product
  Product4 : Product
  Sum5 : Sum  Inputs=|+-
  Sum6 : Sum  Inputs=-++
  chi1 : Integrator  InitialCondition=chi_0
  Y : Outport  VectorParamsAs1DForOutWhenUnconnected=off
  wires:
  lambda/1 -> Math Function1/1, Product3/1, Gain3/1
  Gain3/1 -> Sum5/1
  I/1 -> Gain7/1
  Gain7/1 -> Sum5/2
  Sum5/1 -> Product3/2
  Product3/1 -> Gain8/1
  Math Function1/1 -> Gain9/1
  Gain9/1 -> Product4/2
  chi1/1 -> Y/1, Product4/1
  Product4/1 -> Sum6/1
  v/1 -> Sum6/3
  Gain8/1 -> Sum6/2
  Sum6/1 -> chi1/1

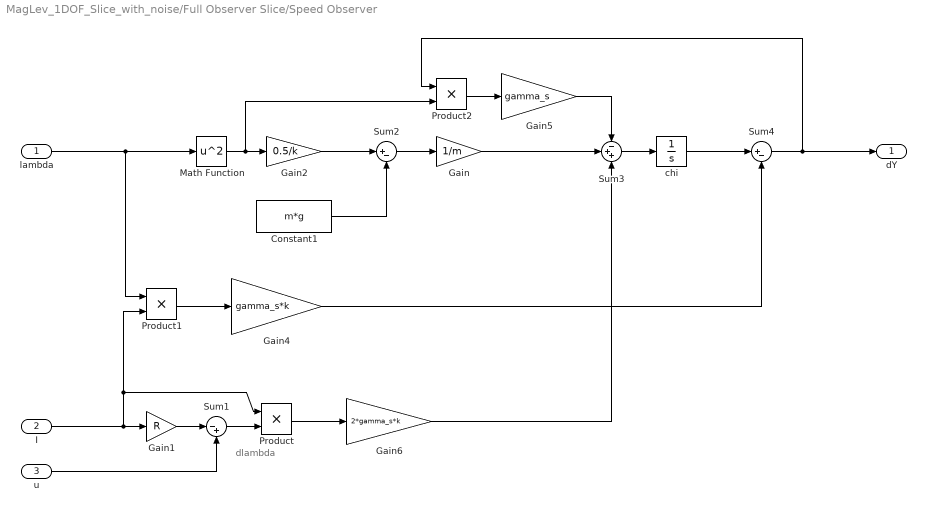
== system MagLev_1DOF_Slice_with_noise/Full Observer Slice/Speed Observer ==
  note: dlambda
  lambda : Inport
  I : Inport  Port=2
  u : Inport  Port=3
  Constant1 : Constant  Value=m*g
  Gain : Gain  Gain=1/m
  Gain1 : Gain  Gain=R
  Gain2 : Gain  Gain=0.5/k
  Gain4 : Gain  Gain=gamma_s*k
  Gain5 : Gain  Gain=gamma_s
  Gain6 : Gain  Gain=2*gamma_s*k
  Math Function : Math  Operator=square  SignedPower=on  SaturateOnIntegerOverflow=on
  Product : Product
  Product1 : Product
  Product2 : Product
  Sum1 : Sum  Inputs=|-+
  Sum2 : Sum  Inputs=|+-
  Sum3 : Sum  Inputs=-++
  Sum4 : Sum  Inputs=|+-
  chi : Integrator
  dY : Outport  VectorParamsAs1DForOutWhenUnconnected=off
  wires:
  u/1 -> Sum1/2
  Gain1/1 -> Sum1/1
  I/1 -> Product1/2, Product/1, Gain1/1
  lambda/1 -> Math Function/1, Product1/1
  Math Function/1 -> Product2/2, Gain2/1
  Sum2/1 -> Gain/1
  Sum1/1 -> Product/2
  Product/1 -> Gain6/1
  Sum3/1 -> chi/1
  chi/1 -> Sum4/1
  Product1/1 -> Gain4/1
  Gain4/1 -> Sum4/2
  Sum4/1 -> Product2/1, dY/1
  Gain/1 -> Sum3/2
  Constant1/1 -> Sum2/2
  Gain2/1 -> Sum2/1
  Product2/1 -> Gain5/1
  Gain5/1 -> Sum3/1
  Gain6/1 -> Sum3/3

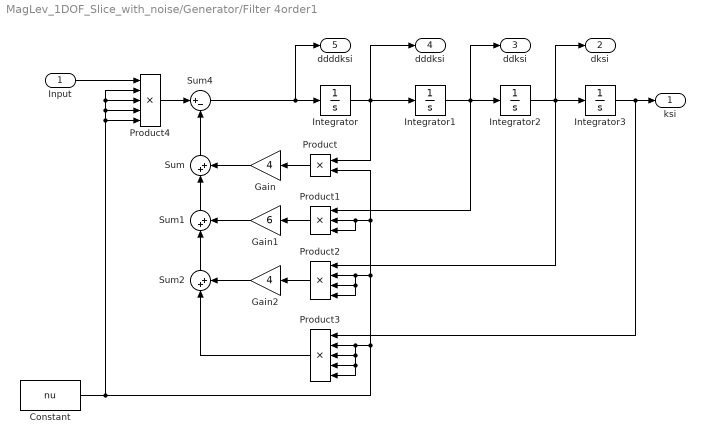
== system MagLev_1DOF_Slice_with_noise/Generator/Filter 4order1 ==
  Input : Inport
  Constant : Constant  Value=nu
  Gain : Gain  Gain=4
  Gain1 : Gain  Gain=6
  Gain2 : Gain  Gain=4
  Integrator{,1..3} (4 alike) : Integrator
  Product : Product  RndMeth=Zero
  Product1 : Product  Inputs=3  RndMeth=Zero
  Product2 : Product  Inputs=4  RndMeth=Zero
  Product3 : Product  Inputs=5  RndMeth=Zero
  Product4 : Product  Inputs=5  RndMeth=Zero
  Sum : Sum  Inputs=|++
  Sum1 : Sum  Inputs=|++
  Sum2 : Sum  Inputs=|++
  Sum4 : Sum  Inputs=|+-
  ksi : Outport  VectorParamsAs1DForOutWhenUnconnected=off
  dksi : Outport  Port=2  VectorParamsAs1DForOutWhenUnconnected=off
  ddksi : Outport  Port=3  VectorParamsAs1DForOutWhenUnconnected=off
  dddksi : Outport  Port=4  VectorParamsAs1DForOutWhenUnconnected=off
  ddddksi : Outport  Port=5  VectorParamsAs1DForOutWhenUnconnected=off
  wires:
  Integrator/1 -> dddksi/1, Product/1, Integrator1/1
  Integrator1/1 -> Integrator2/1, Product1/1, ddksi/1
  Integrator2/1 -> Integrator3/1, Product2/1, dksi/1
  Integrator3/1 -> Product3/1, ksi/1
  Sum4/1 -> Integrator/1, ddddksi/1
  Sum/1 -> Sum4/2
  Sum1/1 -> Sum/1
  Sum2/1 -> Sum1/1
  Product4/1 -> Sum4/1
  Product/1 -> Gain/1
  Product1/1 -> Gain1/1
  Product2/1 -> Gain2/1
  Product3/1 -> Sum2/1
  Constant/1 -> Product4/5, Product4/4, Product4/3, Product4/2, Product3/5, Product3/4, Product3/3, Product3/2, Product2/4, Product2/3, Product2/2, Product1/3, Product1/2, Product/2
  Input/1 -> Product4/1
  Gain/1 -> Sum/2
  Gain1/1 -> Sum1/2
  Gain2/1 -> Sum2/2

== system MagLev_1DOF_Slice_with_noise/regression model/  regression model ==
  v : Inport
  Bus Selector1 : BusSelector  OutputSignals=q1,q2,phi1,phi2,psi,omega1,omega2
  W : Subsystem
  W^2 : Subsystem
  W^3 : Subsystem
  terms of the real q4 : MATLAB Function  TreatAsAtomicUnit=on
  z : Outport  VectorParamsAs1DForOutWhenUnconnected=off
  phi : Outport  Port=2  VectorParamsAs1DForOutWhenUnconnected=off
  wires:
  Bus Selector1/7 -> terms of the real q4/7(omega2)  "<omega2>"
  Bus Selector1/6 -> terms of the real q4/6(omega1)  "<omega1>"
  v/1 -> Bus Selector1/1
  Bus Selector1/1 -> terms of the real q4/1(q1)  "<q1>"
  Bus Selector1/2 -> terms of the real q4/2(q2)  "<q2>"
  Bus Selector1/3 -> terms of the real q4/3(phi1)  "<phi1>"
  Bus Selector1/4 -> terms of the real q4/4(phi2)  "<phi2>"
  Bus Selector1/5 -> terms of the real q4/5(psi)  "<psi>"
  W/1(Out) -> terms of the real q4/8(W1)
  terms of the real q4/3(w1) -> W/1(In)
  terms of the real q4/4(w2) -> W^2/1(In1)
  W^2/1(Out1) -> terms of the real q4/9(W2)
  terms of the real q4/5(w3) -> W^3/1(In1)
  W^3/1(Out1) -> terms of the real q4/10(W3)
  terms of the real q4/1(z) -> z/1
  terms of the real q4/2(phi) -> phi/1

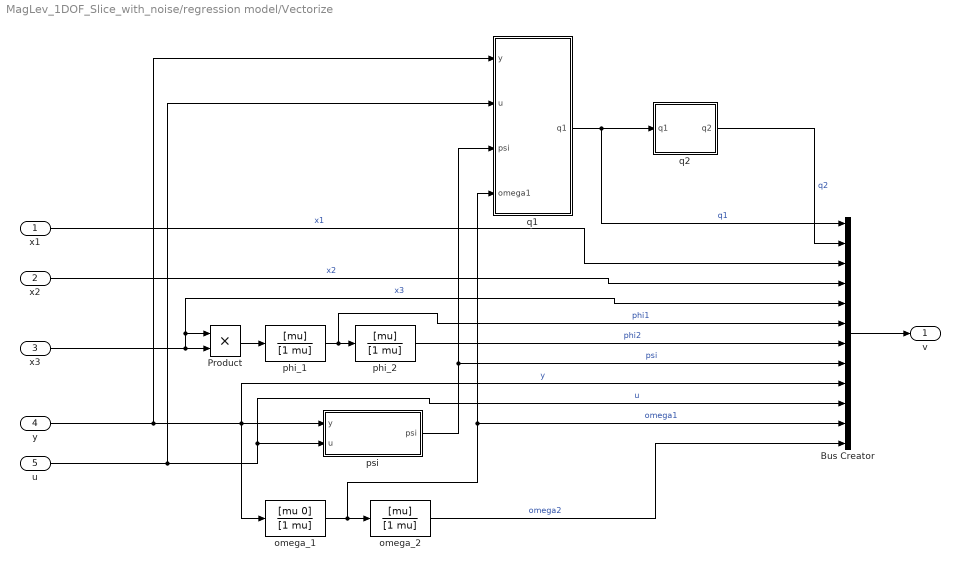
== system MagLev_1DOF_Slice_with_noise/regression model/Vectorize ==
  x1 : Inport
  x2 : Inport  Port=2
  x3 : Inport  Port=3
  y : Inport  Port=4
  u : Inport  Port=5
  Bus Creator : BusCreator  Inputs=12
  Product : Product
  omega_1 : TransferFcn  Numerator=[mu 0]  Denominator=[1 mu]
  omega_2 : TransferFcn  Numerator=[mu]  Denominator=[1 mu]
  phi_1 : TransferFcn  Numerator=[mu]  Denominator=[1 mu]
  phi_2 : TransferFcn  Numerator=[mu]  Denominator=[1 mu]
  psi : Subsystem
  q1 : Subsystem
  q2 : Subsystem
  v : Outport  VectorParamsAs1DForOutWhenUnconnected=off
  wires:
  phi_1/1 -> Bus Creator/6, phi_2/1  "phi1"
  Product/1 -> phi_1/1
  omega_1/1 -> q1/4(omega1), Bus Creator/11, omega_2/1  "omega1"
  Bus Creator/1 -> v/1
  y/1 -> q1/1(y), Bus Creator/9, omega_1/1, psi/1(y)  "y"
  u/1 -> q1/2(u), Bus Creator/10, psi/2(u)  "u"
  x3/1 -> Bus Creator/5, Product/1, Product/2  "x3"
  q1/1(q1) -> q2/1(q1), Bus Creator/1  "q1"
  x1/1 -> Bus Creator/3  "x1"
  x2/1 -> Bus Creator/4  "x2"
  q2/1(q2) -> Bus Creator/2  "q2"
  psi/1(psi) -> q1/3(psi), Bus Creator/8  "psi"
  phi_2/1 -> Bus Creator/7  "phi2"
  omega_2/1 -> Bus Creator/12  "omega2"

== system MagLev_1DOF_Slice_with_noise/regression model1/  regression model ==
  v : Inport
  Bus Selector1 : BusSelector  OutputSignals=q1,q2,phi1,phi2,psi,omega1,omega2
  W : Subsystem
  W^2 : Subsystem
  W^3 : Subsystem
  terms of the real q4 : MATLAB Function  TreatAsAtomicUnit=on
  z : Outport  VectorParamsAs1DForOutWhenUnconnected=off
  phi : Outport  Port=2  VectorParamsAs1DForOutWhenUnconnected=off
  wires:
  Bus Selector1/7 -> terms of the real q4/7(omega2)  "<omega2>"
  Bus Selector1/6 -> terms of the real q4/6(omega1)  "<omega1>"
  v/1 -> Bus Selector1/1
  Bus Selector1/1 -> terms of the real q4/1(q1)  "<q1>"
  Bus Selector1/2 -> terms of the real q4/2(q2)  "<q2>"
  Bus Selector1/3 -> terms of the real q4/3(phi1)  "<phi1>"
  Bus Selector1/4 -> terms of the real q4/4(phi2)  "<phi2>"
  Bus Selector1/5 -> terms of the real q4/5(psi)  "<psi>"
  W/1(Out) -> terms of the real q4/8(W1)
  terms of the real q4/3(w1) -> W/1(In)
  terms of the real q4/4(w2) -> W^2/1(In1)
  W^2/1(Out1) -> terms of the real q4/9(W2)
  terms of the real q4/5(w3) -> W^3/1(In1)
  W^3/1(Out1) -> terms of the real q4/10(W3)
  terms of the real q4/1(z) -> z/1
  terms of the real q4/2(phi) -> phi/1

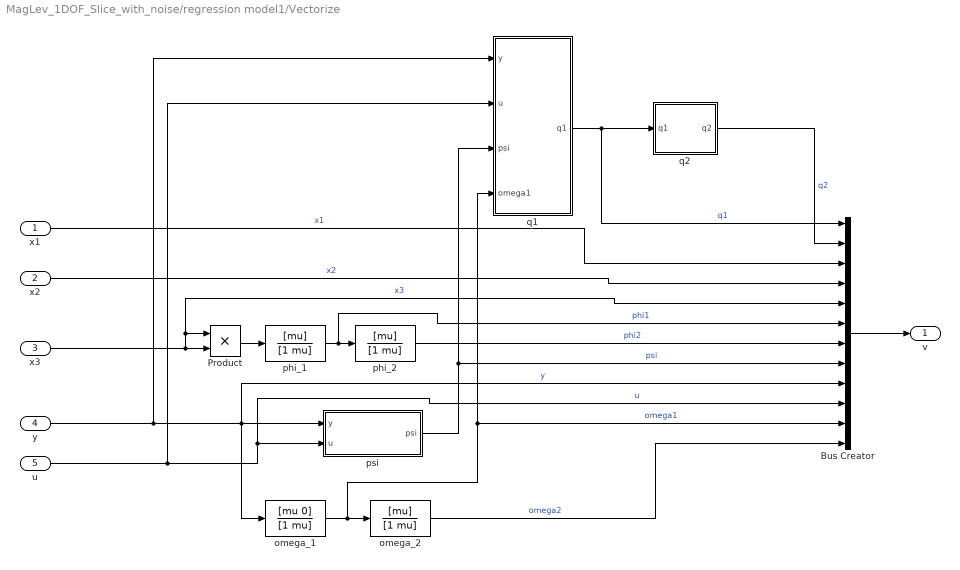
== system MagLev_1DOF_Slice_with_noise/regression model1/Vectorize ==
  x1 : Inport
  x2 : Inport  Port=2
  x3 : Inport  Port=3
  y : Inport  Port=4
  u : Inport  Port=5
  Bus Creator : BusCreator  Inputs=12
  Product : Product
  omega_1 : TransferFcn  Numerator=[mu 0]  Denominator=[1 mu]
  omega_2 : TransferFcn  Numerator=[mu]  Denominator=[1 mu]
  phi_1 : TransferFcn  Numerator=[mu]  Denominator=[1 mu]
  phi_2 : TransferFcn  Numerator=[mu]  Denominator=[1 mu]
  psi : Subsystem
  q1 : Subsystem
  q2 : Subsystem
  v : Outport  VectorParamsAs1DForOutWhenUnconnected=off
  wires:
  phi_1/1 -> Bus Creator/6, phi_2/1  "phi1"
  Product/1 -> phi_1/1
  omega_1/1 -> q1/4(omega1), Bus Creator/11, omega_2/1  "omega1"
  Bus Creator/1 -> v/1
  y/1 -> q1/1(y), Bus Creator/9, omega_1/1, psi/1(y)  "y"
  u/1 -> q1/2(u), Bus Creator/10, psi/2(u)  "u"
  x3/1 -> Bus Creator/5, Product/1, Product/2  "x3"
  q1/1(q1) -> q2/1(q1), Bus Creator/1  "q1"
  x1/1 -> Bus Creator/3  "x1"
  x2/1 -> Bus Creator/4  "x2"
  q2/1(q2) -> Bus Creator/2  "q2"
  psi/1(psi) -> q1/3(psi), Bus Creator/8  "psi"
  phi_2/1 -> Bus Creator/7  "phi2"
  omega_2/1 -> Bus Creator/12  "omega2"

== system MagLev_1DOF_Slice_with_noise/regression model/  regression model/W ==
  In : Inport
  Gain : Gain  Gain=mu
  Gain2 : Gain  Gain=mu
  Integrator : Integrator
  Sum : Sum  Inputs=|+-
  Out : Outport  VectorParamsAs1DForOutWhenUnconnected=off
  wires:
  Gain2/1 -> Out/1
  Sum/1 -> Integrator/1
  Integrator/1 -> Gain/1, Gain2/1
  In/1 -> Sum/1
  Gain/1 -> Sum/2

== system MagLev_1DOF_Slice_with_noise/regression model/  regression model/W^2 ==
  In1 : Inport
  Gain : Gain  Gain=mu
  Gain2 : Gain  Gain=mu
  Gain4 : Gain  Gain=mu^2
  Integrator : Integrator
  Integrator1 : Integrator
  Sum : Sum  Inputs=|+-
  Sum1 : Sum  Inputs=|+-
  Out1 : Outport  VectorParamsAs1DForOutWhenUnconnected=off
  wires:
  In1/1 -> Sum/1
  Gain4/1 -> Out1/1
  Gain2/1 -> Sum1/2
  Integrator/1 -> Gain/1, Sum1/1
  Integrator1/1 -> Gain2/1, Gain4/1
  Sum1/1 -> Integrator1/1
  Gain/1 -> Sum/2
  Sum/1 -> Integrator/1

== system MagLev_1DOF_Slice_with_noise/regression model/  regression model/W^3 ==
  In1 : Inport
  Gain : Gain  Gain=mu
  Gain1 : Gain  Gain=mu
  Gain2 : Gain  Gain=mu
  Gain4 : Gain  Gain=mu^3
  Integrator : Integrator
  Integrator1 : Integrator
  Integrator2 : Integrator
  Sum : Sum  Inputs=|+-
  Sum1 : Sum  Inputs=|+-
  Sum2 : Sum  Inputs=|+-
  Out1 : Outport  VectorParamsAs1DForOutWhenUnconnected=off
  wires:
  Gain4/1 -> Out1/1
  In1/1 -> Sum2/1
  Integrator2/1 -> Gain1/1, Sum/1
  Gain1/1 -> Sum2/2
  Sum2/1 -> Integrator2/1
  Gain2/1 -> Sum1/2
  Integrator/1 -> Gain/1, Sum1/1
  Integrator1/1 -> Gain2/1, Gain4/1
  Sum1/1 -> Integrator1/1
  Gain/1 -> Sum/2
  Sum/1 -> Integrator/1

== system MagLev_1DOF_Slice_with_noise/regression model/Vectorize/psi ==
  y : Inport
  u : Inport  Port=2
  Gain : Gain  Gain=R
  Integrator : Integrator
  Sum : Sum  Inputs=|-+
  psi : Outport  VectorParamsAs1DForOutWhenUnconnected=off
  wires:
  y/1 -> Gain/1
  Gain/1 -> Sum/1
  u/1 -> Sum/2
  Sum/1 -> Integrator/1
  Integrator/1 -> psi/1

== system MagLev_1DOF_Slice_with_noise/regression model/Vectorize/q1 ==
  y : Inport
  u : Inport  Port=2
  psi : Inport  Port=3
  omega1 : Inport  Port=4
  Sum : Sum  Inputs=+-+
  phi_2 : TransferFcn  Numerator=[mu]  Denominator=[1 mu]
  phi_3 : TransferFcn  Denominator=[1 mu]
  terms of the q1 est : MATLAB Function  TreatAsAtomicUnit=on
  q1 : Outport  VectorParamsAs1DForOutWhenUnconnected=off
  wires:
  u/1 -> terms of the q1 est/2(u)
  y/1 -> terms of the q1 est/1(y)
  terms of the q1 est/1(term1) -> phi_2/1
  terms of the q1 est/3(term3) -> phi_3/1
  phi_2/1 -> Sum/1
  terms of the q1 est/2(term2) -> Sum/2
  phi_3/1 -> Sum/3
  omega1/1 -> terms of the q1 est/4(omega1)
  Sum/1 -> q1/1
  psi/1 -> terms of the q1 est/3(psi)

== system MagLev_1DOF_Slice_with_noise/regression model/Vectorize/q2 ==
  q1 : Inport
  Gain1 : Gain  Gain=k*m
  phi_4 : TransferFcn  Numerator=[mu]  Denominator=[1 mu]
  q2 : Outport  VectorParamsAs1DForOutWhenUnconnected=off
  wires:
  q1/1 -> Gain1/1
  Gain1/1 -> phi_4/1
  phi_4/1 -> q2/1

== system MagLev_1DOF_Slice_with_noise/regression model1/  regression model/W ==
  In : Inport
  Gain : Gain  Gain=mu
  Gain2 : Gain  Gain=mu
  Integrator : Integrator
  Sum : Sum  Inputs=|+-
  Out : Outport  VectorParamsAs1DForOutWhenUnconnected=off
  wires:
  Gain2/1 -> Out/1
  Sum/1 -> Integrator/1
  Integrator/1 -> Gain/1, Gain2/1
  In/1 -> Sum/1
  Gain/1 -> Sum/2

== system MagLev_1DOF_Slice_with_noise/regression model1/  regression model/W^2 ==
  In1 : Inport
  Gain : Gain  Gain=mu
  Gain2 : Gain  Gain=mu
  Gain4 : Gain  Gain=mu^2
  Integrator : Integrator
  Integrator1 : Integrator
  Sum : Sum  Inputs=|+-
  Sum1 : Sum  Inputs=|+-
  Out1 : Outport  VectorParamsAs1DForOutWhenUnconnected=off
  wires:
  In1/1 -> Sum/1
  Gain4/1 -> Out1/1
  Gain2/1 -> Sum1/2
  Integrator/1 -> Gain/1, Sum1/1
  Integrator1/1 -> Gain2/1, Gain4/1
  Sum1/1 -> Integrator1/1
  Gain/1 -> Sum/2
  Sum/1 -> Integrator/1

== system MagLev_1DOF_Slice_with_noise/regression model1/  regression model/W^3 ==
  In1 : Inport
  Gain : Gain  Gain=mu
  Gain1 : Gain  Gain=mu
  Gain2 : Gain  Gain=mu
  Gain4 : Gain  Gain=mu^3
  Integrator : Integrator
  Integrator1 : Integrator
  Integrator2 : Integrator
  Sum : Sum  Inputs=|+-
  Sum1 : Sum  Inputs=|+-
  Sum2 : Sum  Inputs=|+-
  Out1 : Outport  VectorParamsAs1DForOutWhenUnconnected=off
  wires:
  Gain4/1 -> Out1/1
  In1/1 -> Sum2/1
  Integrator2/1 -> Gain1/1, Sum/1
  Gain1/1 -> Sum2/2
  Sum2/1 -> Integrator2/1
  Gain2/1 -> Sum1/2
  Integrator/1 -> Gain/1, Sum1/1
  Integrator1/1 -> Gain2/1, Gain4/1
  Sum1/1 -> Integrator1/1
  Gain/1 -> Sum/2
  Sum/1 -> Integrator/1

== system MagLev_1DOF_Slice_with_noise/regression model1/Vectorize/psi ==
  y : Inport
  u : Inport  Port=2
  Gain : Gain  Gain=R
  Integrator : Integrator
  Sum : Sum  Inputs=|-+
  psi : Outport  VectorParamsAs1DForOutWhenUnconnected=off
  wires:
  y/1 -> Gain/1
  Gain/1 -> Sum/1
  u/1 -> Sum/2
  Sum/1 -> Integrator/1
  Integrator/1 -> psi/1

== system MagLev_1DOF_Slice_with_noise/regression model1/Vectorize/q1 ==
  y : Inport
  u : Inport  Port=2
  psi : Inport  Port=3
  omega1 : Inport  Port=4
  Sum : Sum  Inputs=+-+
  phi_2 : TransferFcn  Numerator=[mu]  Denominator=[1 mu]
  phi_3 : TransferFcn  Denominator=[1 mu]
  terms of the q1 est : MATLAB Function  TreatAsAtomicUnit=on
  q1 : Outport  VectorParamsAs1DForOutWhenUnconnected=off
  wires:
  u/1 -> terms of the q1 est/2(u)
  y/1 -> terms of the q1 est/1(y)
  terms of the q1 est/1(term1) -> phi_2/1
  terms of the q1 est/3(term3) -> phi_3/1
  phi_2/1 -> Sum/1
  terms of the q1 est/2(term2) -> Sum/2
  phi_3/1 -> Sum/3
  omega1/1 -> terms of the q1 est/4(omega1)
  Sum/1 -> q1/1
  psi/1 -> terms of the q1 est/3(psi)

== system MagLev_1DOF_Slice_with_noise/regression model1/Vectorize/q2 ==
  q1 : Inport
  Gain1 : Gain  Gain=k*m
  phi_4 : TransferFcn  Numerator=[mu]  Denominator=[1 mu]
  q2 : Outport  VectorParamsAs1DForOutWhenUnconnected=off
  wires:
  q1/1 -> Gain1/1
  Gain1/1 -> phi_4/1
  phi_4/1 -> q2/1

== matlab function MagLev_1DOF_Slice_with_noise/Estimation Slice/Slice algorithm ==
  data: t input; Psi input; zt output; n output; kth output; Z input; R input; Omega_e input; Omega parameter; Omega_p output; dOmega output; gamma_SLICE parameter; epsilon parameter
function [zt, n, kth, Omega_p, dOmega] = fcn(t, Psi, Z, R, Omega_e, Omega, gamma_SLICE, epsilon)

    M = length(Psi);
    ld_columns = zeros(1, M-1); % linear dependent columns index vector
    ln_columns = zeros(1, M); ln_columns(1) = 1;
    K = eye(M, M);
    psil = Psi;

    %% Select linear dependent columns

    ldn = 0;
    lnn = 1;

    for j = 2:M % changed 1
        if (R(j) < epsilon)
            ldn = ldn + 1;
            ld_columns(ldn) = j;
        else
            lnn = lnn + 1;
            ln_columns(lnn) = j;
        end
    end

    if t < 1
        ldn = 0;
        lnn = 6;
        ln_columns = 1:6;
        ld_columns = [];
    end

    n = ldn;
    %% Slice algorithm
    % ldn -- number of linear dependent columns
    % psi1  -- regressor

    for j = 1:ldn
        c = ld_columns(j);                      % Get linear dependent columns index from set
        h = setdiff(1:c-1, ld_columns(1:j-1));  % Diff between subsets
        A = Psi(:, h)\Psi(:, c);                    % Linear combination coeff estimation
        %if cond(Z(:, h)) < 100
        %    A = zeros(size(A));
        %end
        K(h, c) = A;                            % Fill K matrix
        K(c, :) = zeros(1, M);                  % Set row to zero
        psil(:, c) = zeros(M, 1);                 % 
    end

    zt = (psil*K*Omega);
    kth = K(1, :)';
    %zt = 1;
    %kth = 1;

    fcn = @(x) K(1, 1)*x(1) + K(1, 2)*x(1)^2 + K(1, 3)*x(1)^3 + K(1, 4)*x(1)^4 + K(1, 5)*x(1)^5 + K(1, 6)*x(1)^6 - Omega_e(1);
    Omega_p = fzero(fcn, -0.02);
    %th_p = 0;
    
    %% DREM

    %if lnn > 3
    %    lnn = 3;
    %end

    redLPsi = Psi(ln_columns(1:lnn), ln_columns(1:lnn));
    redLZ = Z(ln_columns(1:lnn), 1);

    [s1, s2] = size(redLPsi);
    adjPsi = zeros(size(redLPsi));
    p = 1:s1;

    for i = 1:s1
        for j = 1:s2
            minor = redLPsi(setdiff(p, i), setdiff(p, j));
            adjPsi(j, i) = (-1)^(i + j)*det(minor);
        end
    end

    dOmega = zeros(M, 1);
    dOmega(ln_columns(1:lnn)) = gamma_SLICE*det(redLPsi)*(adjPsi*redLZ - det(redLPsi)*Omega_e(ln_columns(1:lnn)));
%dth = zeros(M, 1);

end

== matlab function MagLev_1DOF_Slice_with_noise/Estimation Slice/QR ==
  data: R output; X input
function R = QR(X)

    Q = zeros(size(X));

    Q(:, 1) = X(:, 1);
    Q(:, 2) = X(:, 2) - dot(X(:, 2), Q(:, 1)) * Q(:, 1)/dot(Q(:, 1), Q(:, 1));

    for i = 3:size(X, 2)
        Q(:, i) = X(:, i) - dot(X(:, i), Q(:, 1)) * Q(:, 1)/dot(Q(:, 1), Q(:, 1));
        for j = 2:i-1
            proj = dot(Q(:, i), Q(:, j)) * Q(:, j)/dot(Q(:, j), Q(:, j));
            Q(:, i) = Q(:, i) - proj;
        end
        Q(:, i) = Q(:, i);
    end

    %R = diag(Q'*X);
    R = diag(Q'*Q);
    R(isnan(R)) = 0;

end

== matlab function MagLev_1DOF_Slice_with_noise/regression model1/  regression model/terms of the real q4 ==
  data: q1 input; q2 input; phi1 input; phi2 input; psi input; omega1 input; omega2 input; W1 input size=10; W2 input size=6; W3 input size=2; k parameter; g parameter; m parameter; z output size=1; phi output size=6; w1 output size=10; w2 output size=6; lambda_0 parameter; w3 output; mu parameter
function [z, phi, w1, w2, w3] = fcn( q1, q2, phi1, phi2, psi, omega1, omega2, W1, W2, W3, k, g, m, lambda_0, mu)

theta = lambda_0;

psi1 = psi;
psi2 = psi1^2;

w1psi1 = W1(1);
w1psi2 = W1(2);
w1psi1w1psi1 = W1(3);
w1psi1w1psi2 = W1(4);
w1psi1w2psi1 = W1(5);
w1psi1w2psi2 = W1(6);
w1a1w1psi1 = W1(7);
w1a1w1psi2 = W1(8);
w1a1w2psi1 = W1(9);
w1a1w2psi2 = W1(10);

w2psi1 = W2(1);
w2psi2 = W2(2);
w2psi1w1psi1 = W2(3);
w2psi1w1psi2 = W2(4);
w2a1w1psi1 = W2(5);
w2a1w1psi2 = W2(6);

w3psi1 = W3(1);
w3psi2 = W3(2);

a1 = psi2 - 2*m*g*k;
psi1w1psi1 = psi1*w1psi1;
psi1w1psi2 = psi1*w1psi2;
psi1w2psi1 = psi1*w2psi1;
psi1w2psi2 = psi1*w2psi2;
a1w1psi1 = a1*w1psi1;
a1w1psi2 = a1*w1psi2;
a1w2psi1 = a1*w2psi1;
a1w2psi2 = a1*w2psi2;

w1 = [
  psi1;
  psi2;
  psi1w1psi1;
  psi1w1psi2;
  psi1w2psi1;
  psi1w2psi2;
  a1w1psi1;
  a1w1psi2;
  a1w2psi1;
  a1w2psi2
];

w2 = [
  psi1;
  psi2;
  psi1w1psi1;
  psi1w1psi2;
  a1w1psi1;
  a1w1psi2
];

w3 = [
  psi1;
  psi2;
];

% z = 2*k*mu*(k*m*q1*phi2 - q2*phi1) ...
%     + w2psi2*w1a1w1psi2 ...
%     - w1psi2*w1a1w2psi2 ...
%     - w1psi2*w2a1w1psi2;
% 
% phi1 =  ( omega1*w2psi2 - omega2*w1psi2 )*2*k^2*m*mu ...
%     - ( 2*w2psi1*w1a1w1psi2 + w2psi2*(2*w1psi1w1psi2 + 2*w1a1w1psi1) ) ...
%     + ( 2*w1psi1*w1a1w2psi2 + w1psi2*(2*w1psi1w2psi2 + 2*w1a1w2psi1) ) ...
%     + (2*w1psi1*w2a1w1psi2 + w1psi2*(2*w2psi1w1psi2 + 2*w2a1w1psi1));
%     
% phi2 = ( omega1*w2psi1 - omega2*w1psi1 )*4*k^2*m*mu ...
%     - ( w1a1w1psi2 + 4*w2psi1*(w1psi1w1psi2 + w1a1w1psi1) + w2psi2*(w1psi2 - 2*m*g*k + w2psi2 + 4*w1psi1w1psi1) ) ...
%     + ( w1a1w2psi2 + 4*w1psi1*(w1psi1w2psi2 + w1a1w2psi1) + w1psi2*(w1psi2 - 2*m*g*k + w3psi2 + 4*w1psi1w2psi1) ) ...
%     + (w2a1w1psi2 + 4*w1psi1*(w2psi1w1psi2 + w2a1w1psi1) + w1psi2*(w2psi2 - 2*m*g*k + w3psi2 + 4*w2psi1w1psi1));
% 
% phi3 = ( omega1 - omega2 )*2*k^2*m*mu ...
%     - ( 2*w1psi1w1psi2 + 2*w1a1w1psi1 + 2*w2psi1*(w1psi2 - 2*m*g*k + w2psi2 + 4*w1psi1w1psi1) + 2*w2psi2*(w1psi1 + w2psi1) ) ...
%     + ( 2*w1psi1w2psi2 + 2*w1a1w2psi1 + 2*w1psi1*(w1psi2 - 2*m*g*k + w3psi2 + 4*w1psi1w2psi1) + 2*w1psi2*(w1psi1 + w3psi1) ) ...
%     + (2*w2psi1w1psi2 + 2*w2a1w1psi1 + 2*w1psi1*(w2psi2 - 2*m*g*k + w3psi2 + 4*w2psi1w1psi1) + 2*w1psi2*(w2psi1 + w3psi1));
% 
% phi4 = - ( w1psi2 - 2*m*g*k + w2psi2 + 4*w1psi1w1psi1 + 4*w2psi1*(w1psi1 + w2psi1) + w2psi2 ) ...
%     + ( w1psi2 - 2*m*g*k + w3psi2 + 4*w1psi1w2psi1 + 4*w1psi1*(w1psi1 + w3psi1) + w1psi2 ) ...
%     + (w2psi2 - 2*m*g*k + w3psi2 + 4*w2psi1w1psi1 + 4*w1psi1*(w2psi1 + w3psi1) + w1psi2);

z = 2*k*mu*(k*m*q1*phi2 - q2*phi1) ...
    - w1psi2*(w1a1w2psi2 + w2a1w1psi2) ...
    + w2psi2*w1a1w1psi2;

phi1 =  ( omega1*w2psi2 - omega2*w1psi2 )*2*k^2*m*mu ...
    + 2*w1psi1*(w1a1w2psi2 + w2a1w1psi2) ...
    + 2*w1psi2*(w1psi1w2psi2 + w1a1w2psi1 + w2psi1w1psi2 + w2a1w1psi1) ...
    - 2*w2psi1*w1a1w1psi2 ...
    - 2*w2psi2*(w1psi1w1psi2 + w1a1w1psi1);
    
phi2 = ( omega1*w2psi1 - omega2*w1psi1 )*4*k^2*m*mu ...
    + 2*m*g*k*(w2psi2 - 2*w1psi2) ...
    + (w1psi2)^2 - (w2psi2)^2 ...
    + 4*w1psi1*(w1psi1w2psi2 + w1a1w2psi1 + w2psi1w1psi2 + w2a1w1psi1) ...
    + 2*w1psi2*(w3psi2 + 2*w1psi1w2psi1 + 2*w2psi1w1psi1) ...
    - 4*w2psi1*(w1psi1w1psi2 + w1a1w1psi1) ...
    - w1a1w1psi2 + w1a1w2psi2 ...
    + w2a1w1psi2 ...
    - 4*w2psi2*w1psi1w1psi1;

phi3 = ( omega1 - omega2 )*2*k^2*m*mu ...
    + 4*m*g*k*(w2psi1 - 2*w1psi1)  ...
    + 4*w1psi1*(w1psi2 + w3psi2 + 2*w1psi1w2psi1 + 2*w2psi1w1psi1) ...
    + 4*w1psi2*w3psi1 ...
    - 4*w2psi1*( w2psi2 + 2*w1psi1w1psi1) ...
    - 2*w1psi1w1psi2 + 2*w1psi1w2psi2+ 2*w2psi1w1psi2 ...
    - 2*w1a1w1psi1+ 2*w1a1w2psi1 + 2*w2a1w1psi1;

phi4 = - 2*m*g*k + 2*w1psi2 - w2psi2 + 2*w3psi2 - 4*w2psi1*w2psi1 ...
    + 4*w1psi1*w1psi1 + 8*w1psi1*w3psi1 ...
    - 4*w1psi1w1psi1 + 4*w1psi1w2psi1 ...
    + 4*w2psi1w1psi1;

phi5 = - 2*w2psi1 + 4*w3psi1 + 4*w1psi1;

phi6 = 1;

phi = [
    phi1;
    phi2;
    phi3;
    phi4;
    phi5;
    phi6
];

== matlab function MagLev_1DOF_Slice_with_noise/regression model1/Vectorize/q1/terms of the q1 est ==
  data: y input; u input; psi input; omega1 input; R parameter; term1 output; term2 output; term3 output
function [term1, term2, term3] = fcn( y, u, psi, omega1, R )

term1 = y*(u - R*y);
term2 = psi*omega1;
term3 = (u - R*y)*omega1;
